simulink model "chapter10"  (R2015a)
settings: Solver=ode45  StartTime=0.0  StopTime=2  RelTol=1e-3
settings Model: Creator=Anu  LastModifiedBy=Anu

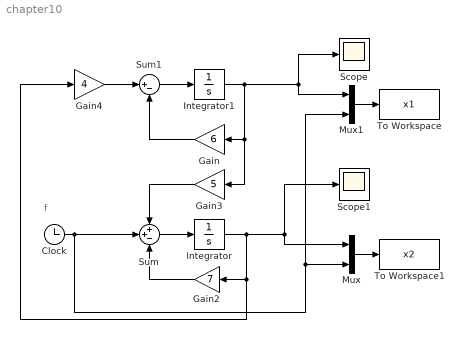
== system chapter10 ==
  note: f
  Clock : Clock
  Gain : Gain  Gain=6
  Gain2 : Gain  Gain=7
  Gain3 : Gain  Gain=5
  Gain4 : Gain  Gain=4
  Integrator : Integrator
  Integrator1 : Integrator
  Mux : Mux  Inputs=2
  Mux1 : Mux  Inputs=2
  Scope : Scope
  Scope1 : Scope
  Sum : Sum  Inputs=++-
  Sum1 : Sum  Inputs=|+-
  To Workspace : ToWorkspace  VariableName=x1  SampleTime=-1
  To Workspace1 : ToWorkspace  VariableName=x2  SampleTime=-1
  wires:
  Gain4/1 -> Sum1/1
  Sum1/1 -> Integrator1/1
  Integrator1/1 -> Mux1/1, Scope/1, Gain3/1, Gain/1
  Gain/1 -> Sum1/2
  Gain3/1 -> Sum/1
  Clock/1 -> Sum/2, Mux/2, Mux1/2
  Sum/1 -> Integrator/1
  Integrator/1 -> Gain4/1, Gain2/1, Mux/1, Scope1/1
  Gain2/1 -> Sum/3
  Mux/1 -> To Workspace1/1
  Mux1/1 -> To Workspace/1
